simulink model "tilting_of_a_drone"  (R2022a)
settings: Solver=VariableStepAuto  StartTime=0.0  StopTime=5  RelTol=1e-3
settings Model: Creator=siddh  LastModifiedBy=siddh

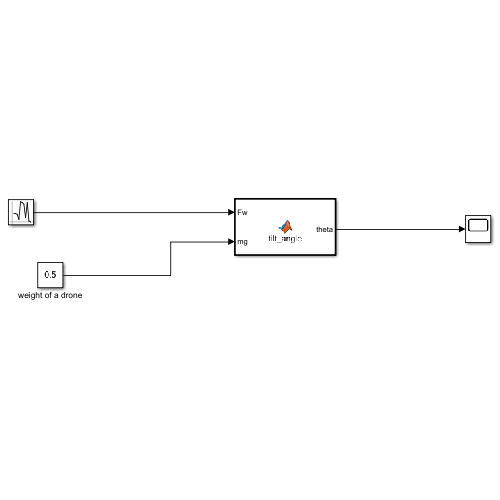
[thumbnail: Simulink's stored preview of the top-level diagram]
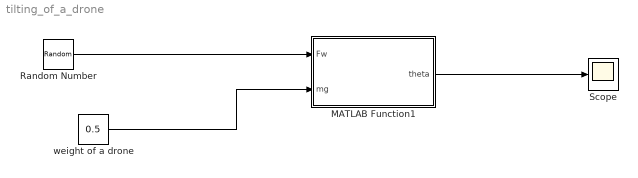
== system tilting_of_a_drone ==
  MATLAB Function1 : MATLAB Function  TreatAsAtomicUnit=on
  Random Number : RandomNumber  Mean=1  SampleTime=0.1
  Scope : Scope
  weight of a drone : Constant  Value=0.5
  wires:
  weight of a drone/1 -> MATLAB Function1/2(mg)
  MATLAB Function1/1(theta) -> Scope/1
  Random Number/1 -> MATLAB Function1/1(Fw)

== matlab function tilting_of_a_drone/MATLAB Function1 ==
  data: Fw input; theta output; mg input
function theta = tilt_angle(Fw,mg)

% Fr*sin(theta) = mg
% Fr*cos(theta) = Fw
% tan(theta) = mg/Fw

theta = atand(mg/Fw);

end
